simulink model "motor_modell"  (R2024a)
settings: Solver=VariableStepAuto  StartTime=0.0  StopTime=20  RelTol=1e-3
model workspace (MAT data in the model file):
  J = 0.00038
  K = 0.028
  L = 0.0001
  R = 5
settings Model: Creator=janho  LastModifiedBy=janho

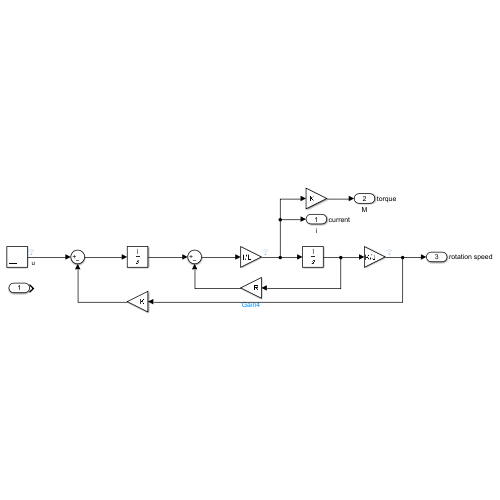
[thumbnail: Simulink's stored preview of the top-level diagram]
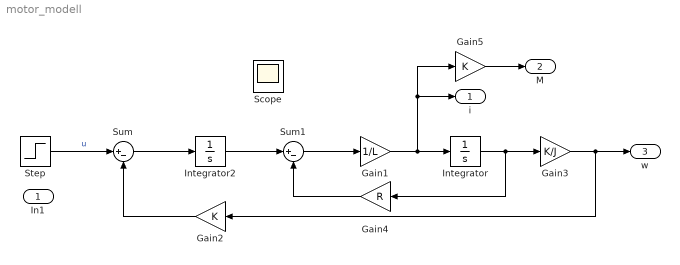
== system motor_modell ==
  In1 : Inport
  Gain1 : Gain  Gain=1/L
  Gain2 : Gain  Gain=K
  Gain3 : Gain  Gain=K/J
  Gain4 : Gain  Gain=R
  Gain5 : Gain  Gain=K
  Integrator : Integrator
  Integrator2 : Integrator
  Step : Step  Time=0  After=10  SampleTime=0
  Sum : Sum  Inputs=|+-
  Sum1 : Sum  Inputs=|+-
  i : Outport  SignalName=current
  M : Outport  Port=2  SignalName=torque
  w : Outport  Port=3  SignalName=rotation speed
  Scope : Scope
  wires:
  Gain5/1 -> M/1
  Sum1/1 -> Gain1/1
  Step/1 -> Sum/1  "u"
  Gain1/1 -> Integrator/1, i/1, Gain5/1
  Sum/1 -> Integrator2/1
  Integrator2/1 -> Sum1/1
  Gain2/1 -> Sum/2
  Gain4/1 -> Sum1/2
  Integrator/1 -> Gain3/1, Gain4/1
  Gain3/1 -> w/1, Gain2/1
